simulink model "lab_part2_withGivenModel"  (R2022a)
settings: Solver=ode45  StartTime=0.0  StopTime=3  MaxStep=0.001  RelTol=1e-3
model workspace (MAT data in the model file):
  a = 2.5
values from neighbouring files (symbols this model uses):
  zeta = .6    (= 0.6)    [init.m]    (also in part3_plot.m)
settings Model: Creator=zhong  LastModifiedBy=zhong
settings DataIOCC: ReturnWorkspaceOutputs=off

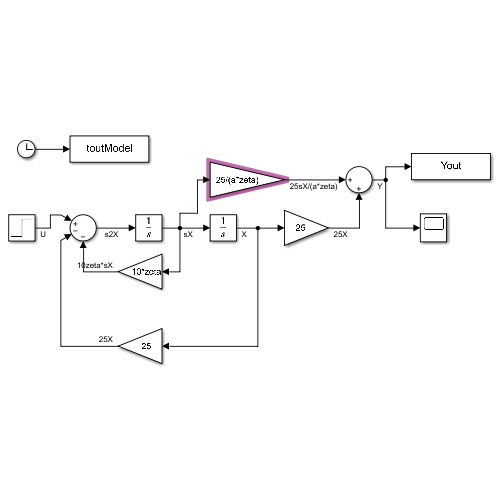
[thumbnail: Simulink's stored preview of the top-level diagram]
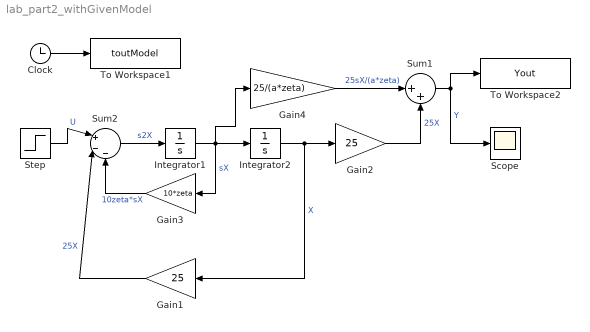
== system lab_part2_withGivenModel ==
  Clock : Clock
  Gain1 : Gain  Gain=25
  Gain2 : Gain  Gain=25
  Gain3 : Gain  Gain=10*zeta
  Gain4 : Gain  Gain=25/(a*zeta)
  Integrator1 : Integrator
  Integrator2 : Integrator
  Scope : Scope
  Step : Step  Time=0  SampleTime=0
  Sum1 : Sum  Inputs=|++
  Sum2 : Sum  Inputs=|+--
  To Workspace1 : ToWorkspace  VariableName=toutModel  SampleTime=-1
  To Workspace2 : ToWorkspace  VariableName=Yout  SampleTime=-1
  wires:
  Integrator1/1 -> Gain4/1, Gain3/1, Integrator2/1  "sX"
  Sum2/1 -> Integrator1/1  "s2X"
  Integrator2/1 -> Gain1/1, Gain2/1  "X"
  Sum1/1 -> To Workspace2/1, Scope/1  "Y"
  Gain2/1 -> Sum1/2  "25X"
  Gain4/1 -> Sum1/1  "25sX/(a*zeta)"
  Step/1 -> Sum2/1  "U"
  Gain3/1 -> Sum2/3  "10zeta*sX"
  Gain1/1 -> Sum2/2  "25X"
  Clock/1 -> To Workspace1/1
